simulink model "rts_project_accel"  (R2024b)
settings: Solver=FixedStepAuto  StartTime=0.0  StopTime=10  FixedStep=0.05  RelTol=1e-3  EnableMultiTasking=on
libraries: arduinolib x3, arduinosensorlib x2, eeGeneralControl x1, slpidlib x1
settings Model: ExtModeTrigDuration=2  Creator=Asus  LastModifiedBy=Asus
settings SolverCC: AutoInsertRateTranBlk=on
settings DataIOCC: ReturnWorkspaceOutputs=off
settings OptimizationCC: EnhancedBackFolding=on  PassReuseOutputArgsAs=Individual arguments  ZeroExternalMemoryAtStartup=off  ZeroInternalMemoryAtStartup=off  MaxStackSize=64  OptimizeBlockOrder=speed  DifferentSizesBufferReuse=on  OptimizationCustomize=off  EfficientTunableParamExpr=on
settings DebuggingCC: ParameterTunabilityLossMsg=error
settings HardwareCC: ProdBitPerInt=16  ProdBitPerPointer=16  ProdBitPerSizeT=16  ProdBitPerPtrDiffT=16  ProdLargestAtomicFloat=None  ProdWordSize=8  ProdHWDeviceType=Atmel->AVR
settings SFSimCC: MATLABDynamicMemAlloc=off
settings RTWCC: Description=Embedded Coder  SystemTargetFile=ert.tlc  HardwareBoard=Arduino Mega 2560  TLCOptions="-aInlineSetEventsForThisBaseRateFcn=TLC_FALSE -aSuppressMultiTaskScheduler=TLC_FALSE   -aRateBasedStepFcn=1"  TemplateMakefile=ert_default_tmf  Toolchain=Arduino AVR  BuildConfiguration=Faster Runs
settings CodeAppCC: ForceParamTrailComments=on  IgnoreCustomStorageClasses=off  OperatorAnnotations=on  SimulinkDataObjDesc=on  SFDataObjDesc=on  InsertBlockDesc=on
settings ERTTargetCC: SupportContinuousTime=on  SupportVariableSizeSignals=on  ExtModeTransport=3  ExtModeStaticAlloc=on  ExtModeAutomaticAllocSize=off  ExtModeStaticAllocSize=2048  ExtModeMexFile=ext_xcp  ExtModeIntrfLevel=Level2 - Open  InlinedParameterPlacement=Hierarchical

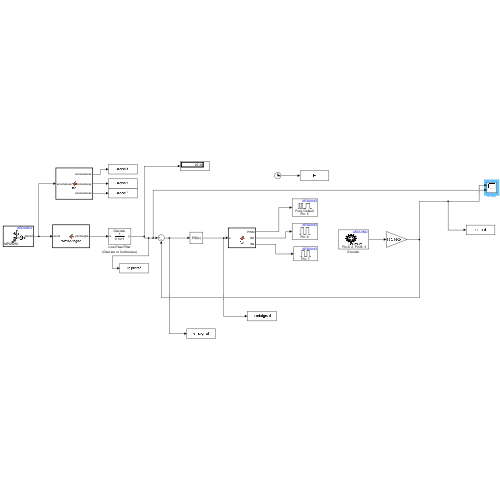
[thumbnail: Simulink's stored preview of the top-level diagram]
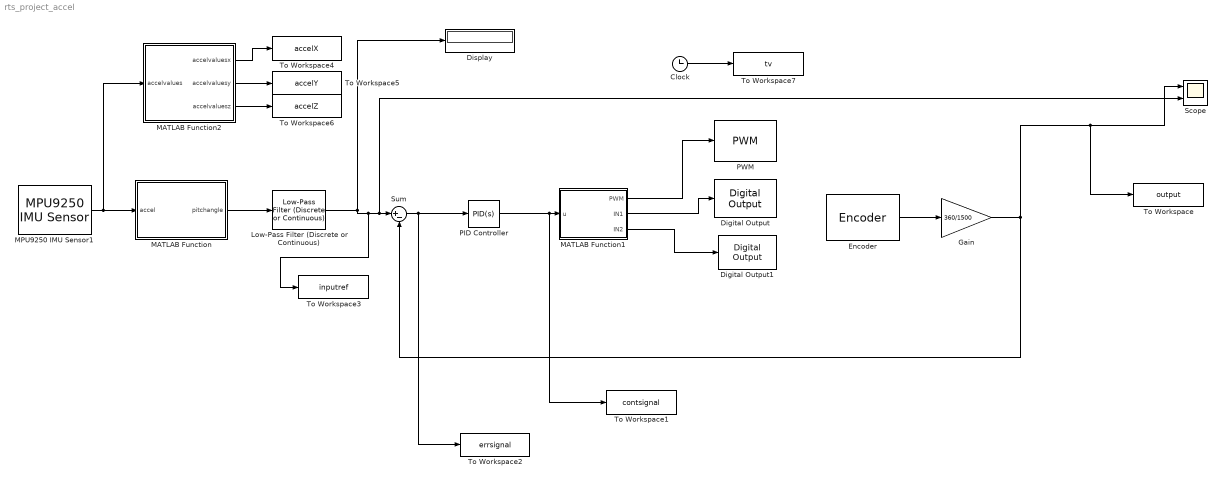
== system rts_project_accel ==
  Clock : Clock
  Digital Output : arduinolib/Digital Output  pinNumber=6  Direction=output  blockPlatform=arduino
      settings: SourceProductName=Common
  Digital Output1 : arduinolib/Digital Output  pinNumber=7  Direction=output  blockPlatform=arduino
      settings: SourceProductName=Common
  Display : Display
  Encoder : arduinosensorlib/Encoder  InputA=2  InputB=3  Mode=No reset  SampleTime=-1
      settings: SourceProductName=Sensors
  Gain : Gain  Gain=360/1500
  Low-Pass Filter (Discrete or Continuous) : eeGeneralControl/Low-Pass Filter (Discrete or Continuous)  K=1  T=0.1  B=90  A=-90  init_option=Inherited from block input  x0=0  Ts=-1
  MATLAB Function : MATLAB Function  TreatAsAtomicUnit=on
  MATLAB Function1 : MATLAB Function  TreatAsAtomicUnit=on
  MATLAB Function2 : MATLAB Function  TreatAsAtomicUnit=on
  MPU9250 IMU Sensor1 : arduinosensorlib/MPU9250 IMU Sensor  I2CModule=0  SlaveAddress=0x68  Accel=on  AngularRate=off  Ak8963Field=off  Temperature=off  Status=off  EulerAngles=off  Quat=off  Timestamp=off  AccelRange=2G  Acceldlpf=1046 Hz  GyroRange=250 dps  Gyrodlpf=250 Hz  DmpOdr=200 Hz  spf=1  SampleTime=-1  QueueSizeFactor=1
      settings: SourceProductName=Sensors
  PID Controller : slpidlib/PID Controller  Controller=PID  Form=Parallel  TimeDomain=Continuous-time  UseExternalTs=off  SampleTime=-1  IntegratorMethod=Forward Euler  FilterMethod=Forward Euler  ControllerParametersSource=internal  P=0.465  I=0.48954  UseKiTs=off  D=0.0005  UseExternalDerivativeSource=off  N=0  UseFilter=on  TunerSelectOption=Transfer Function Based (PID Tuner App)  InitialConditionSource=internal  InitialConditionForIntegrator=0  InitialConditionForFilter=0  DifferentiatorICPrevScaledInput=0  ExternalReset=none  TrackingMode=off  Kt=1  LimitOutput=off  SatLimitsSource=internal  UpperSaturationLimit=inf  LowerSaturationLimit=-inf  LinearizeAsGain=on  AntiWindupMode=none  Kb=1  LimitIntegrator=off  UpperIntegratorSaturationLimit=inf  LowerIntegratorSaturationLimit=-inf  POutMin=[]  POutMax=[]  IOutMin=[]  IOutMax=[]  DOutMin=[]  DOutMax=[]  NOutMin=[]  NOutMax=[]  SumOutMin=[]  SumOutMax=[]  SaturationOutMin=[]  SaturationOutMax=[]  PParamMin=[]  PParamMax=[]  IParamMin=[]  IParamMax=[]  DParamMin=[]  DParamMax=[]  NParamMin=[]  NParamMax=[]  KbParamMin=[]  KbParamMax=[]  KtParamMin=[]  KtParamMax=[]  KbOutMin=[]  KbOutMax=[]  KtOutMin=[]  KtOutMax=[]  IntegratorOutMin=[]  IntegratorOutMax=[]  FilterOutMin=[]  FilterOutMax=[]  SumI1OutMin=[]  SumI1OutMax=[]  SumI2OutMin=[]  SumI2OutMax=[]  SumI3OutMin=[]  SumI3OutMax=[]  SumI4OutMin=[]  SumI4OutMax=[]  SumDOutMin=[]  SumDOutMax=[]  DifferentiatorOutMin=[]  DifferentiatorOutMax=[]  FilterDiffOutCoefMin=[]  FilterDiffOutCoefMax=[]  ReciprocalOutMin=[]  ReciprocalOutMax=[]  SumDenOutMin=[]  SumDenOutMax=[]  SumNumOutMin=[]  SumNumOutMax=[]  DivideOutMin=[]  DivideOutMax=[]  UdiffTsProdOutMin=[]  UdiffTsProdOutMax=[]  NTsProdOutMin=[]  NTsProdOutMax=[]  UintegralTsProdOutMin=[]  UintegralTsProdOutMax=[]  UngainTsProdOutMin=[]  UngainTsProdOutMax=[]  ClampingZeroOutDataTypeStr=Inherit: Inherit via back propagation  ClampingZeroOutMin=[]  ClampingZeroOutMax=[]  FilterDenConstantOutDataTypeStr=Inherit: Inherit via back propagation  FilterDenConstantOutMin=[]  FilterDenConstantOutMax=[]  PCopyOutDataTypeStr=Inherit: Inherit via back propagation  PCopyOutMin=[]  PCopyOutMax=[]  NCopyOutDataTypeStr=Inherit: Inherit via back propagation  NCopyOutMin=[]  NCopyOutMax=[]  IntegratorContinuousStateAttributes=''  IntegratorStateMustResolveToSignalObject=off  IntegratorRTWStateStorageClass=Auto  FilterContinuousStateAttributes=''  FilterStateMustResolveToSignalObject=off  FilterRTWStateStorageClass=Auto  ParallelPVariant=InternalParameters  IdealPVariant=Disabled  IVariant=InternalParameters  DVariant=InternalParameters  IntegratorVariant=Continuous  SatVariant=Disabled  AWVariant=Passthrough  PCopyVariant=Disabled  TRVariant=Disabled  FdbkBlocksVariant=Forward  IdealPFdbkVariant=Disabled  SatFdbkVariant=Disabled  DerivativeFilterVariant=ContFilter  NVariant=InternalParameters  NCopyVariant=Disabled  FilterICVariant=InternalICsFilter  IntegratorICVariant=InternalICs  ExternalResetVariant=Disabled  TRSumVariant=Passthrough  SumFdbkVariant=Disabled  SumVariant=Sum_PID  TsampFilterVariant=InternalTs  TsampNgainVariant=Passthrough  TsampIntegralVariant=Disabled_SignalSpec  ExternalSaturationOutDataTypeStr=Inherit: Same as second input  DerivativeSourceVariant=ErrorSignal  PreIntVariant=InternalPreInt
  PWM : arduinolib/PWM  pinNumber=5  frequencyType=Default  desiredFrequency=490.2  achievableFrequency=490.2
      settings: SourceProductName=Common
  Scope : Scope  NumInputPorts=2
  Sum : Sum  Inputs=|+-
  To Workspace : ToWorkspace  VariableName=output  SampleTime=-1
      settings: Save2DSignal=2-D array (concatenate along first dimension)
  To Workspace1 : ToWorkspace  VariableName=contsignal  SampleTime=-1
      settings: Save2DSignal=2-D array (concatenate along first dimension)
  To Workspace2 : ToWorkspace  VariableName=errsignal  SampleTime=-1
      settings: Save2DSignal=2-D array (concatenate along first dimension)
  To Workspace3 : ToWorkspace  VariableName=inputref  SampleTime=-1
      settings: Save2DSignal=2-D array (concatenate along first dimension)
  To Workspace4 : ToWorkspace  VariableName=accelX  SampleTime=-1
      settings: Save2DSignal=2-D array (concatenate along first dimension)
  To Workspace5 : ToWorkspace  VariableName=accelY  SampleTime=-1
      settings: Save2DSignal=2-D array (concatenate along first dimension)
  To Workspace6 : ToWorkspace  VariableName=accelZ  SampleTime=-1
      settings: Save2DSignal=2-D array (concatenate along first dimension)
  To Workspace7 : ToWorkspace  VariableName=tv  SampleTime=-1
      settings: Save2DSignal=2-D array (concatenate along first dimension)
  wires:
  Sum/1 -> PID Controller/1, To Workspace2/1
  Encoder/1 -> Gain/1
  MPU9250 IMU Sensor1/1 -> MATLAB Function/1(accel), MATLAB Function2/1(accelvalues)
  MATLAB Function1/1(PWM) -> PWM/1
  MATLAB Function1/2(IN1) -> Digital Output/1
  MATLAB Function1/3(IN2) -> Digital Output1/1
  MATLAB Function2/2(accelvaluesy) -> To Workspace5/1
  MATLAB Function2/3(accelvaluesz) -> To Workspace6/1
  MATLAB Function2/1(accelvaluesx) -> To Workspace4/1
  Clock/1 -> To Workspace7/1
  Gain/1 -> Sum/2, To Workspace/1, Scope/1
  PID Controller/1 -> To Workspace1/1, MATLAB Function1/1(u)
  MATLAB Function/1(pitchangle) -> Low-Pass Filter (Discrete or Continuous)/1
  Low-Pass Filter (Discrete or Continuous)/1 -> To Workspace3/1, Scope/2, Sum/1, Display/1

== matlab function rts_project_accel/MATLAB Function ==
  data: accel input; pitchangle output
function pitchangle = convToAngles(accel)


% Accel verilerini ayır
accel_x = accel(1);
accel_y = accel(2);
accel_z = accel(3);


% Pitch açısı hesaplama (derece cinsinden)
pitchangle = atan2(-accel_x, sqrt(accel_y^2 + accel_z^2)) * (180 / pi);
end

== matlab function rts_project_accel/MATLAB Function2 ==
  data: accelvalues input; accelvaluesx output; accelvaluesy output; accelvaluesz output
function [accelvaluesx, accelvaluesy,accelvaluesz]= fcn(accelvalues)
accelvaluesx=accelvalues(1)
accelvaluesy=accelvalues(2)
accelvaluesz=accelvalues(3)

end

== matlab function rts_project_accel/MATLAB Function1 ==
  data: u input; PWM output; IN1 output; IN2 output
function [PWM,IN1,IN2] = fcn(u)
PWM=abs(u);
if u<0
    IN1=1;
    IN2=0;
elseif u>0
    IN1=0;
    IN2=1;
else
    IN1=0;
    IN2=0;
end
